simulink model "dcMotor_fourQChopper"  (R2021a)
settings: Solver=VariableStepAuto  StartTime=0.0  StopTime=3  FixedStep=1e-5  MaxStep=1e-6  RelTol=1e-3  EnableMultiTasking=on
values from neighbouring files (symbols this model uses):
  D1 = 240/Vdc    (= 0.8)    [fourQchopper_script.m]
  rated_torque = rated_power/rated_speed    (= 20.3454584681)    [fourQchopper_script.m]
  Ts = 1/f_switching    (= 0.000166666666667)    [fourQchopper_script.m]
  Vdc = 300    [fourQchopper_script.m]
  Vtri = 1    [fourQchopper_script.m]
libraries: spsMosfetLib x4, spsDCVoltageSourceLib x2, spsDCMachineLib x1, spsGroundLib x1, simulink x1, spsVoltageMeasurementLib x1, spspowerguiLib x1
settings Model: Creator=dinesh  LastModifiedBy=USER
settings SolverCC: AlgebraicLoopSolver=TrustRegion
settings DataIOCC: LimitDataPoints=on  SaveFormat=Array  SignalLoggingSaveFormat=ModelDataLogs  SignalLoggingName=sigsOut
settings DebuggingCC: SaveWithParameterizedLinksMsg=none  SignalResolutionControl=TryResolveAllWithWarning  MultiTaskDSMMsg=warning  MultiTaskCondExecSysMsg=none  SFMachineParentedDataDiag=warning
settings HardwareCC: ProdBitPerPointer=32  ProdBitPerSizeT=32  ProdBitPerPtrDiffT=32  ProdLargestAtomicFloat=None  ProdIntDivRoundTo=Undefined  ProdEndianess=Unspecified  ProdWordSize=32  ProdHWDeviceType=32-bit Generic  TargetUnknown=on
settings ModelReferenceCC: PropagateSignalLabelsOutOfModel=off
settings GRTTargetCC: CombineOutputUpdateFcns=off  GRTInterface=on
settings ConfigComp: CovMetricSettings=dw  CovSaveCumulativeToWorkspaceVar=on  CovSaveSingleToWorkspaceVar=on

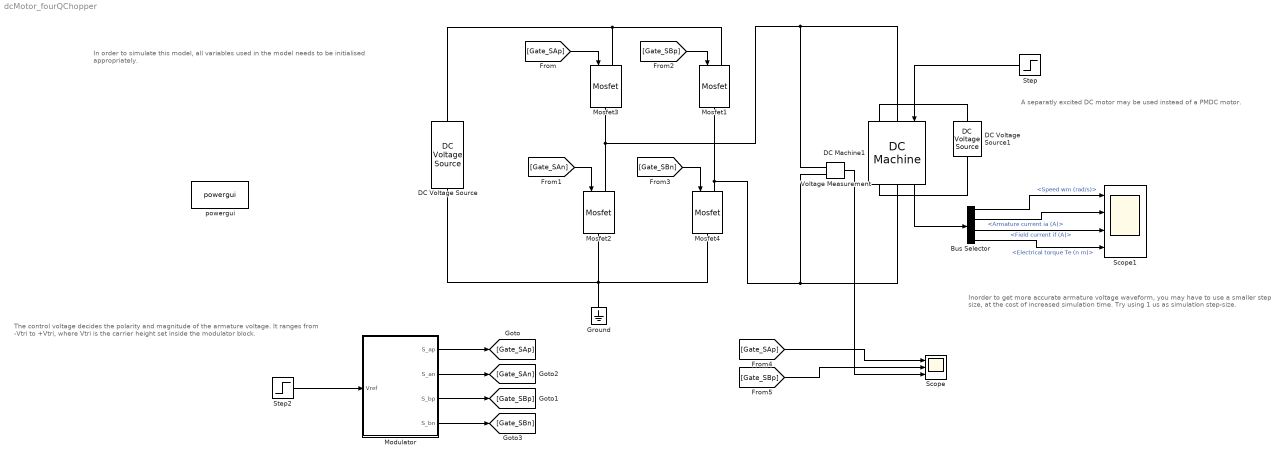
== system dcMotor_fourQChopper ==
  note: A separatly excited DC motor may be used instead of a PMDC motor.
  note: The control voltage decides the polarity and magnitude of the
      | armature voltage. It ranges from -Vtri to +Vtri, where Vtri is the carrier height set inside the modulator block.
  note: Inorder to get more accurate armature voltage
      | waveform, you may have to use a smaller step size, at the cost of increased simulation time. Try using 1 us as
      | simulation step-size.
  note: In order to simulate this model, all variables used in the model needs to be initialised appropriately.
  Bus Selector : BusSelector  OutputSignals=Speed wm (rad/s),Armature current ia (A),Field current if (A),Electrical torque Te (n m)
  DC Machine1 : spsDCMachineLib/DC Machine  PresetModel=01: 5HP 240V 1750RPM Field:300V  MechanicalLoad=Torque TL  FieldType=Wound  ShowDetailedParameters=on  MeasurementBus=off  RLa=[2.581 0.028]  RLf=[281.2 156]  Laf=0.9483  MachineConstant=Torque constant (N.m/A)  Ke=1.8  Kt=1.8  J=0.02215  Bm=0.002953  Tf=0.5161  w0=1  Ifinit=1.06685633001422  TsPowergui=0  TsBlock=-1
  DC Voltage Source : spsDCVoltageSourceLib/DC Voltage Source  Amplitude=Vdc  Measurements=None
  DC Voltage Source1 : spsDCVoltageSourceLib/DC Voltage Source  Amplitude=300  Measurements=None
  Ground : spsGroundLib/Ground  LConnTagsString=a
  Modulator : Subsystem
  Mosfet{1..4} (4 alike) : spsMosfetLib/Mosfet  Ron=0.1  Lon=0  Rd=0.01  Vfd=0  IC=0  Rs=1e5  Cs=inf  Measurements=off
  Scope : Scope  NumInputPorts=3
  Scope1 : Scope  NumInputPorts=4
  Step : Step  After=rated_torque  SampleTime=0
  Step2 : Step  Time=2  Before=D1  After=-D1  SampleTime=0
  Voltage Measurement : spsVoltageMeasurementLib/Voltage Measurement  PhasorSimulation=off  OutputType=Complex  PSBequivalent=0
  powergui : spspowerguiLib/powergui  Priority=1  SimulationMode=Continuous  SampleTime=50e-6  frequency=60  Iterations=50  frequencyindice=0  Pbase=100e6  ErrMax=1e-4  UnitsV=kV  UnitsW=MW  buscounter=0  FunctionMessages=off  echomessages=off  EnableUseOfTLC=off  CurrentSourceSwitches=off  DisableSnubberDevices=off  DisableRonSwitches=off  DisableVfSwitches=off  DisplayEquations=off  AutomaticDiscreteSolvers=off  SolverType=Tustin/Backward Euler (TBE)  Interpol=off  ExternalGateDelay=off  methode=off  Ts=100  x0status=blocks  SPID=on  SwTol=0  HookPort=off  NonlinearTolerance=1e-4  nMaxIteration=100  ContinueOnMaxIteration=off  RestoreLinks=warning  ResistiveCurrentMeasurement=off  Frange=[0:2:500]  Ylog=off  Xlog=on  ShowGrid=off  save=off  variable=ZData  structure=0  ZoomFFT=off  StartTime=0.0  cycles=1  DisplayStyle=1  fundamental=60  FreqAxis=off  MaxFrequency=1000  frequencyindicesteady=1  RmsSteady=1  display=off
  wires:
  [Gate_SAn] -> Mosfet2/1
  [Gate_SAp] -> Mosfet3/1
  [Gate_SBp] -> Mosfet1/1
  [Gate_SBn] -> Mosfet4/1
  Modulator/1(S_ap) -> [Gate_SAp]
  Modulator/3(S_bp) -> [Gate_SBp]
  Step/1 -> DC Machine1/1
  DC Machine1/1 -> Bus Selector/1
  Step2/1 -> Modulator/1(Vref)
  [Gate_SBp] -> Scope/2
  Voltage Measurement/1 -> Scope/3
  [Gate_SAp] -> Scope/1
  Modulator/2(S_an) -> [Gate_SAn]
  Modulator/4(S_bn) -> [Gate_SBn]
  Bus Selector/1 -> Scope1/1  "<Speed wm (rad/s)>"
  Bus Selector/2 -> Scope1/2  "<Armature current ia (A)>"
  Bus Selector/3 -> Scope1/3  "<Field current if (A)>"
  Bus Selector/4 -> Scope1/4  "<Electrical torque Te (n m)>"
  connections:
  DC Machine1/LConn1 -- Mosfet2/LConn1 -- Mosfet3/RConn1 -- Voltage Measurement/LConn1
  DC Voltage Source/RConn1 -- Mosfet3/LConn1 -- Mosfet1/LConn1
  DC Voltage Source/LConn1 -- Ground/LConn1 -- Mosfet4/RConn1 -- Mosfet2/RConn1
  Mosfet4/LConn1 -- Mosfet1/RConn1 -- DC Machine1/RConn1 -- Voltage Measurement/LConn2
  DC Machine1/LConn2 -- DC Voltage Source1/LConn1
  DC Machine1/RConn2 -- DC Voltage Source1/RConn1

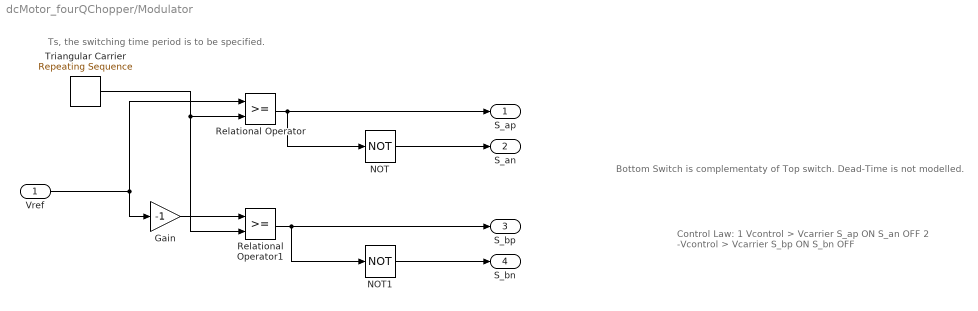
== system dcMotor_fourQChopper/Modulator ==
  note: Control Law:
      |
      | 1
      | Vcontrol > Vcarrier
      | S_ap
      | ON
      | S_an
      | OFF
      |
      | 2
      | -Vcontrol > Vcarrier
      | S_bp
      | ON
      | S_bn
      | OFF
  note: Ts, the switching time period is to be specified.
  note: Bottom Switch is complementaty of Top switch. Dead-Time is not modelled.
  Vref : Inport
  Gain : Gain  Gain=-1  SaturateOnIntegerOverflow=on  OutDataTypeStr=Inherit: Same as input  ParamDataTypeStr=Inherit: Same as input
  NOT : Logic  Operator=NOT  IconShape=distinctive  AllPortsSameDT=off  OutDataTypeStr=boolean
  NOT1 : Logic  Operator=NOT  IconShape=distinctive  AllPortsSameDT=off  OutDataTypeStr=boolean
  Relational Operator : RelationalOperator  RndMeth=Nearest
  Relational Operator1 : RelationalOperator  RndMeth=Nearest
  Triangular Carrier : simulink/Sources/Repeating Sequence  rep_seq_t=[0 0.5*Ts Ts]  rep_seq_y=[Vtri -Vtri Vtri]
  S_ap : Outport
  S_an : Outport  Port=2
  S_bp : Outport  Port=3
  S_bn : Outport  Port=4
  wires:
  Vref/1 -> Relational Operator/1, Gain/1
  Relational Operator/1 -> NOT/1, S_ap/1
  Triangular Carrier/1 -> Relational Operator/2, Relational Operator1/2
  Relational Operator1/1 -> NOT1/1, S_bp/1
  NOT/1 -> S_an/1
  NOT1/1 -> S_bn/1
  Gain/1 -> Relational Operator1/1
